simulink model "abe_x_theta_simple"  (R2022a)
settings: Solver=VariableStepAuto  StartTime=0.0  StopTime=50  RelTol=1e-3
libraries: simulink x1
settings Model: Creator=Abraham  LastModifiedBy=Abraham

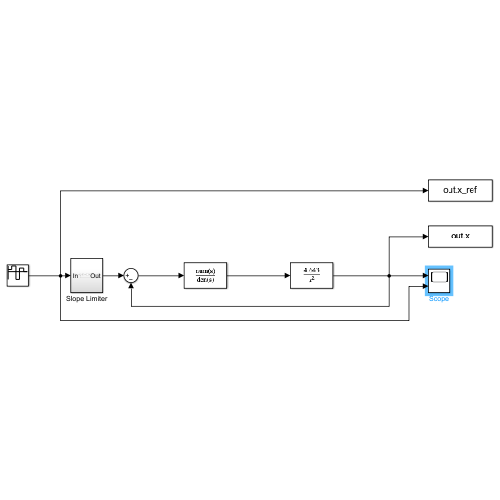
[thumbnail: Simulink's stored preview of the top-level diagram]
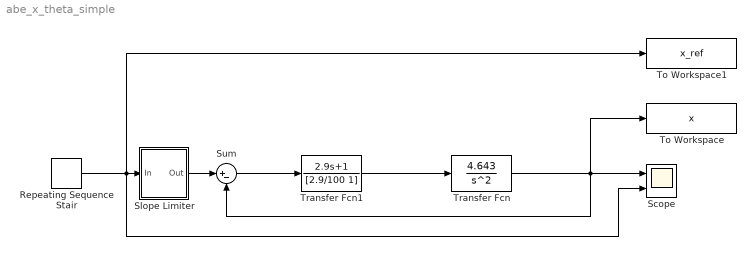
== system abe_x_theta_simple ==
  Repeating Sequence Stair : simulink/Sources/Repeating Sequence Stair  OutValues=[5 15 -20 10 0]  tsamp=10  OutMin=[]  OutMax=[]  OutDataTypeStr=double  OutputDataTypeScalingMode=double  OutDataType=fixdt(0,8)  ConRadixGroup=Best Precision: Vector-wise  OutScaling=2^-12
  Scope : Scope  NumInputPorts=2
  Slope Limiter : Subsystem
  Sum : Sum  Inputs=|+-
  To Workspace : ToWorkspace  VariableName=x  SaveFormat=Timeseries  SampleTime=-1
  To Workspace1 : ToWorkspace  VariableName=x_ref  SaveFormat=Timeseries  SampleTime=-1
  Transfer Fcn : TransferFcn  Numerator=[4.643]  Denominator=[1 0 0]
  Transfer Fcn1 : TransferFcn  Numerator=[2.9 1]  Denominator=[2.9/100 1]
  wires:
  Transfer Fcn/1 -> To Workspace/1, Scope/1, Sum/2
  Slope Limiter/1(Out) -> Sum/1
  Repeating Sequence Stair/1 -> To Workspace1/1, Scope/2, Slope Limiter/1(In)
  Sum/1 -> Transfer Fcn1/1
  Transfer Fcn1/1 -> Transfer Fcn/1

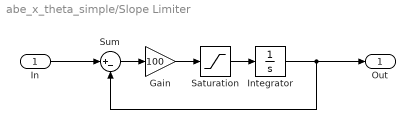
== system abe_x_theta_simple/Slope Limiter ==
  In : Inport
  Gain : Gain  Gain=100
  Integrator : Integrator
  Saturation : Saturate  UpperLimit=10  LowerLimit=-10
  Sum : Sum  Inputs=|+-
  Out : Outport
  wires:
  Integrator/1 -> Out/1, Sum/2
  Gain/1 -> Saturation/1
  Saturation/1 -> Integrator/1
  Sum/1 -> Gain/1
  In/1 -> Sum/1
